simulink model "Proposed DTC"  (R2022a)
settings: Solver=ode1  StartTime=0.0  StopTime=Inf  FixedStep=Ts  RelTol=1e-3  EnableMultiTasking=on
PostLoadFcn:
  | , if any(exist('dsrtsu_mdlpostloadfcn', 'file') ~= 0), dsrtsu_mdlpostloadfcn('Execute', bdroot); end,
InitFcn:
  | , if any(exist('rtifpga_mdlclblib', 'file') ~= 0), rtifpga_mdlclblib('Init', bdroot); end,
undefined symbols (not defined in the file): P, Ts
libraries: rtilib1104 x15, rtitasklib x1
(part 2 of 2)

== matlab function Proposed DTC/Controller/MATLAB Function2 ==
  data: del_psi input; V output; del_T input; n input; psi_s1 input; is_1 input; psi_s_ref input; T_ref input; Vdc input; Ts input; w input; Dfinal output
function [V,Dfinal] = fcn(del_psi,del_T,n,psi_s1,is_1,psi_s_ref,T_ref,Vdc,Ts,w)
Dfinal=1;
T_max=1; T_min=-1;
psi_max=0.01; psi_min=-0.01;
Ls=0.022;
psi_r=0.5;
V=1;
V1=2/5*Vdc*(1.6180+1j*0);
V2=2/5*Vdc*(1.3090+1j*0.9511);
V3=2/5*Vdc*(0.5+1j*1.5390);
V4=2/5*Vdc*(-0.5+1j*1.5390);
V5=2/5*Vdc*(-1.3090+1j*0.9511);
V6=2/5*Vdc*(-1.6180+1j*0);
V7=2/5*Vdc*(-1.3090-1j*0.9511);
V8=2/5*Vdc*(-0.5-1j*1.5390);
V9=2/5*Vdc*(0.5-1j*1.5390);
V10=2/5*Vdc*(1.3090-1j*0.9511);
V11=2/5*Vdc*(1+1j*0);
V12=2/5*Vdc*(0.8090+1j*0.5878);
V13=2/5*Vdc*(0.3090+1j*0.9511);
V14=2/5*Vdc*(-0.3090+1j*0.9511);
V15=2/5*Vdc*(-0.8090+1j*0.5878);
V16=2/5*Vdc*(-1+1j*0);
V17=2/5*Vdc*(-0.8090-1j*0.5878);
V18=2/5*Vdc*(-0.3090-1j*0.9511);
V19=2/5*Vdc*(0.3090-1j*0.9511);
V20=2/5*Vdc*(0.8090-1j*0.5878);
V21=2/5*Vdc*(0.6180+1j*0);
V22=2/5*Vdc*(0.5+1j*0.3633);
V23=2/5*Vdc*(0.1910+1j*0.5878);
V24=2/5*Vdc*(-0.1910+1j*0.5878);
V25=2/5*Vdc*(-0.5+1j*0.3633);
V26=2/5*Vdc*(-0.6180+1j*0);
V27=2/5*Vdc*(-0.5-1j*0.3633);
V28=2/5*Vdc*(-0.1910-1j*0.5878);
V29=2/5*Vdc*(0.1910-1j*0.5878);
V30=2/5*Vdc*(0.5-1j*0.3633);
V31=0;
v=[V1 V2 V3 V4 V5 V6 V7 V8 V9 V10 V11 V12 V13 V14 V15 V16 V17 V18 V19 V20 V21 V22 V23 V24 V25 V26 V27 V28 V29 V30 V31];
% states=[1 1 0 0 1;
%         1 1 0 0 0;
%         1 1 1 0 0;
%         0 1 1 0 0;
%         0 1 1 1 0;
%         0 0 1 1 0;
%         0 0 1 1 1;
%         0 0 0 1 1;
%         1 0 0 1 1;
%         1 0 0 0 1;
%         1 0 0 0 0;
%         1 1 1 0 1;
%         0 1 0 0 0;
%         1 1 1 1 0;
%         0 0 1 0 0;
%         0 1 1 1 1;
%         0 0 0 1 0;
%         1 0 1 1 1;
%         0 0 0 0 1;
%         1 1 0 1 1;
%         0 1 0 0 1;
%         1 1 0 1 0;
%         1 0 1 0 0;
%         0 1 1 0 1;
%         0 1 0 1 0;
%         1 0 1 1 0;
%         0 0 1 0 1;
%         0 1 0 1 1;
%         1 0 0 1 0;
%         1 0 1 0 1;
%         0 0 0 0 0];
VT=0;Vpsi=0;
kk=0;
persistent dec k D_psi D_T x y 
if isempty(dec), dec = 0; end
if isempty(k), k = 0; end
if isempty(D_psi), D_psi = 0; end
if isempty(D_T), D_T = 0; end
if isempty(x), x = 31; end
if isempty(y), y = 31; end

if del_T>T_max
    del_T=1;
elseif del_T<T_min
    del_T=-1;
else
    del_T=0;
end
if del_psi>psi_max
    del_psi=1;
elseif del_psi<psi_min
    del_psi=-1;
else
    del_psi=0;
end
%     D=1;
if abs(w)>157.07
    D=abs(w)/314;
else
    D=0.5;
end
% High speed of operation
if((abs(w)>=0&&abs(w)<=314))
if dec==0
    if del_T==1
        if n==1 || n==2
            VT=v(4);x=4;
        elseif n==3 || n==4
            VT=v(5);x=5;
        elseif n==5 || n==6
            VT=v(6);x=6;
        elseif n==7 || n==8
            VT=v(7);x=7;
        elseif n==9 || n==10
            VT=v(8);x=8;
        elseif n==11 || n==12
            VT=v(9);x=9;
        elseif n==13 || n==14
            VT=v(10);x=10;
        elseif n==15 || n==16
            VT=v(1);x=1;
        elseif n==17 || n==18
            VT=v(2);x=2;
        elseif n==19 || n==20
            VT=v(3);x=3;
        end
    elseif del_T==-1
        if n==1 || n==2
            VT=v(9);x=9;
        elseif n==3 || n==4
            VT=v(10);x=10;
        elseif n==5 || n==6
            VT=v(1);x=1;
        elseif n==7 || n==8
            VT=v(2);x=2;
        elseif n==9 || n==10
            VT=v(3);x=3;
        elseif n==11 || n==12
            VT=v(4);x=4;
        elseif n==13 || n==14
            VT=v(5);x=5;
        elseif n==15 || n==16
            VT=v(6);x=6;
        elseif n==17 || n==18
            VT=v(7);x=7;
        elseif n==19 || n==20
            VT=v(8);x=8;
        end
    end
    if del_psi==1
        if n==2 || n==3
            Vpsi=v(2);y=2;
            VT=v(4);x=4;
            if del_T==-1
                VT=v(10);x=10;
            end
        elseif n==4 || n==5
            Vpsi=v(3);y=3;
            VT=v(5);x=5;
            if del_T==-1
                VT=v(1);x=1;
            end
        elseif n==6 || n==7
            Vpsi=v(4);y=4;
            VT=v(6);x=6;
            if del_T==-1
                VT=v(2);x=2;
            end
        elseif n==8 || n==9
            Vpsi=v(5);y=5;
            VT=v(7);x=7;
            if del_T==-1
                VT=v(3);x=3;
            end
        elseif n==10 || n==11
            Vpsi=v(6);y=6;
            VT=v(8);x=8;
            if del_T==-1
                VT=v(4);x=4;
            end
        elseif n==12 || n==13
            Vpsi=v(7);y=7;
            VT=v(9);x=9;
            if del_T==-1
                VT=v(5);x=5;
            end
        elseif n==14 || n==15
            Vpsi=v(8);y=8;
            VT=v(10);x=10;
            if del_T==-1
                VT=v(6);x=6;
            end
        elseif n==16 || n==17
            Vpsi=v(9);y=9;
            VT=v(1);x=1;
            if del_T==-1
                VT=v(7);x=7;
            end
        elseif n==18 || n==19
            Vpsi=v(10);y=10;
            VT=v(2);x=2;
            if del_T==-1
                VT=v(8);x=8;
            end
        elseif n==20 || n==1
            Vpsi=v(1);y=1;
            VT=v(3);x=3;
            if del_T==-1
                VT=v(9);x=9;
            end
        end
    elseif del_psi==-1
        if n==2 || n==3
            Vpsi=v(7);y=7;
            VT=v(5);x=5;
            if del_T==-1
                VT=v(9);x=9;
            end
        elseif n==4 || n==5
            Vpsi=v(8);y=8;
            VT=v(6);x=6;
            if del_T==-1
                VT=v(10);x=10;
            end
        elseif n==6 || n==7
            Vpsi=v(9);y=9;
            VT=v(7);x=7;
            if del_T==-1
                VT=v(1);x=1;
            end
        elseif n==8 || n==9
            Vpsi=v(10);y=10;
            VT=v(8);x=8;
            if del_T==-1
                VT=v(2);x=2;
            end
        elseif n==10 || n==11
            Vpsi=v(1);y=1;
            VT=v(9);x=9;
            if del_T==-1
                VT=v(3);x=3;
            end
        elseif n==12 || n==13
            Vpsi=v(2);y=2;
            VT=v(10);x=10;
            if del_T==-1
                VT=v(4);x=4;
            end
        elseif n==14 || n==15
            Vpsi=v(3);y=3;
            VT=v(1);x=1;
            if del_T==-1
                VT=v(5);x=5;
            end
         elseif n==16 || n==17
            Vpsi=v(4);y=4;
            VT=v(2);x=2;
            if del_T==-1
                VT=v(6);x=6;
            end
         elseif n==18 || n==19
            Vpsi=v(5);y=5;
            VT=v(3);x=3;
            if del_T==-1
                VT=v(7);x=7;
            end
         elseif n==20 || n==1
            Vpsi=v(6);y=6;
            VT=v(4);x=4;
            if del_T==-1
                VT=v(8);x=8;
            end
        end
    elseif del_psi==0
        y=x;
    end
    if del_T==0
        VT=0;Vpsi=0;x=31;y=31;
    end    
    M=abs(VT)*Ts*sin(angle(VT)-angle(psi_s1));    
    Q=Ls*(T_ref/(5*psi_r)-abs(is_1)*sin(angle(is_1)-angle(psi_s1)));    
    if del_T==0
        D_psi=0;
        D_T=0;
    end
    dec=1;
    if del_psi==0
        D_T=0.5*Q/M;        
        D_psi=D_T;
    else
        D_T=D;
        kk=1;
        k=1;
    end
    V=x;
    Dfinal=D_T;
end
k=k+1;
if k==2
    k=0;
    dec=0;
end
if dec==0 && kk==0
    if del_T==1
        if n==1 || n==2
            VT=v(4);x=4;
        elseif n==3 || n==4
            VT=v(5);x=5;
        elseif n==5 || n==6
            VT=v(6);x=6;
        elseif n==7 || n==8
            VT=v(7);x=7;
        elseif n==9 || n==10
            VT=v(8);x=8;
        elseif n==11 || n==12
            VT=v(9);x=9;
        elseif n==13 || n==14
            VT=v(10);x=10;
        elseif n==15 || n==16
            VT=v(1);x=1;
        elseif n==17 || n==18
            VT=v(2);x=2;
        elseif n==19 || n==20
            VT=v(3);x=3;
        end
    elseif del_T==-1
        if n==1 || n==2
            VT=v(9);x=9;
        elseif n==3 || n==4
            VT=v(10);x=10;
        elseif n==5 || n==6
            VT=v(1);x=1;
        elseif n==7 || n==8
            VT=v(2);x=2;
        elseif n==9 || n==10
            VT=v(3);x=3;
        elseif n==11 || n==12
            VT=v(4);x=4;
        elseif n==13 || n==14
            VT=v(5);x=5;
        elseif n==15 || n==16
            VT=v(6);x=6;
        elseif n==17 || n==18
            VT=v(7);x=7;
        elseif n==19 || n==20
            VT=v(8);x=8;
        end
    end

    if del_psi==1
        if n==2 || n==3
            Vpsi=v(2);k=0;
        elseif n==4 || n==5
            Vpsi=v(3);k=0;
        elseif n==6 || n==7
            Vpsi=v(4);k=0;
        elseif n==8 || n==9
            Vpsi=v(5);k=0;
        elseif n==10 || n==11
            Vpsi=v(6);k=0;
        elseif n==12 || n==13
            Vpsi=v(7);k=0;
        elseif n==14 || n==15
            Vpsi=v(8);k=0;
        elseif n==16 || n==17
            Vpsi=v(9);k=0;
        elseif n==18 || n==19
            Vpsi=v(10);k=0;
        elseif n==20 || n==1
            Vpsi=v(1);k=0;    
        end
    elseif del_psi==0
        if n==2 || n==3
            Vpsi=v(7);k=0;
        elseif n==4 || n==5
            Vpsi=v(8);k=0;
        elseif n==6 || n==7
            Vpsi=v(9);k=0;
        elseif n==8 || n==9
            Vpsi=v(10);k=0;
        elseif n==10 || n==11
            Vpsi=v(1);k=0;
        elseif n==12 || n==13
            Vpsi=v(2);k=0;
        elseif n==14 || n==15
            Vpsi=v(3);k=0;
        elseif n==16 || n==17
            Vpsi=v(4);k=0;
        elseif n==18 || n==19
            Vpsi=v(5);k=0;
        elseif n==20 || n==1
            Vpsi=v(6);k=0;
        end
    end
    if del_T==0
        VT=0;Vpsi=0;x=31;
    end
    A=abs(VT)*Ts*cos(angle(VT)-angle(psi_s1));
    B=abs(Vpsi)*Ts*cos(angle(Vpsi)-angle(psi_s1));
    M=abs(VT)*Ts*sin(angle(VT)-angle(psi_s1));
    N=abs(Vpsi)*Ts*sin(angle(Vpsi)-angle(psi_s1));
    K=psi_s_ref-abs(psi_s1);
    Q=Ls*(T_ref/(5*psi_r)-abs(is_1)*sin(angle(is_1)-angle(psi_s1)));
    V=y;
    Dfinal=D_psi;
end
% Medium speed of operation
% elseif(abs(w)>100 && abs(w)<=200)
% if dec==0
%     if del_T==1
%         if n==1 || n==2
%             VT=v(14);x=14;
%         elseif n==3 || n==4
%             VT=v(15);x=15;
%         elseif n==5 || n==6
%             VT=v(16);x=16;
%         elseif n==7 || n==8
%             VT=v(17);x=17;
%         elseif n==9 || n==10
%             VT=v(18);x=18;
%         elseif n==11 || n==12
%             VT=v(19);x=19;
%         elseif n==13 || n==14
%             VT=v(20);x=20;
%         elseif n==15 || n==16
%             VT=v(11);x=11;
%         elseif n==17 || n==18
%             VT=v(12);x=12;
%         elseif n==19 || n==20
%             VT=v(13);x=13;
%         end
%     elseif del_T==-1
%         if n==1 || n==2
%             VT=v(19);x=19;
%         elseif n==3 || n==4
%             VT=v(20);x=20;
%         elseif n==5 || n==6
%             VT=v(11);x=11;
%         elseif n==7 || n==8
%             VT=v(12);x=12;
%         elseif n==9 || n==10
%             VT=v(13);x=13;
%         elseif n==11 || n==12
%             VT=v(14);x=14;
%         elseif n==13 || n==14
%             VT=v(15);x=15;
%         elseif n==15 || n==16
%             VT=v(16);x=16;
%         elseif n==17 || n==18
%             VT=v(17);x=17;
%         elseif n==19 || n==20
%             VT=v(18);x=18;
%         end
%     end
%     if del_psi==1
%         if n==2 || n==3
%             Vpsi=v(12);y=12;
%             VT=v(14);x=14;
%             if del_T==-1
%                 VT=v(20);x=20;
%             end
%         elseif n==4 || n==5
%             Vpsi=v(13);y=13;
%             VT=v(15);x=15;
%             if del_T==-1
%                 VT=v(11);x=11;
%             end
%         elseif n==6 || n==7
%             Vpsi=v(14);y=14;
%             VT=v(16);x=16;
%             if del_T==-1
%                 VT=v(12);x=12;
%             end
%         elseif n==8 || n==9
%             Vpsi=v(15);y=15;
%             VT=v(17);x=17;
%             if del_T==-1
%                 VT=v(13);x=13;
%             end
%         elseif n==10 || n==11
%             Vpsi=v(16);y=16;
%             VT=v(18);x=18;
%             if del_T==-1
%                 VT=v(14);x=14;
%             end
%         elseif n==12 || n==13
%             Vpsi=v(17);y=17;
%             VT=v(19);x=19;
%             if del_T==-1
%                 VT=v(15);x=15;
%             end
%         elseif n==14 || n==15
%             Vpsi=v(18);y=18;
%             VT=v(20);x=20;
%             if del_T==-1
%                 VT=v(16);x=16;
%             end
%         elseif n==16 || n==17
%             Vpsi=v(19);y=19;
%             VT=v(11);x=11;
%             if del_T==-1
%                 VT=v(17);x=17;
%             end
%         elseif n==18 || n==19
%             Vpsi=v(20);y=20;
%             VT=v(12);x=12;
%             if del_T==-1
%                 VT=v(18);x=18;
%             end
%         elseif n==20 || n==1
%             Vpsi=v(11);y=11;
%             VT=v(13);x=13;
%             if del_T==-1
%                 VT=v(19);x=19;
%             end
%         end
%     elseif del_psi==-1
%         if n==2 || n==3
%             Vpsi=v(17);y=17;
%             VT=v(15);x=15;
%             if del_T==-1
%                 VT=v(19);x=19;
%             end
%         elseif n==4 || n==5
%             Vpsi=v(18);y=18;
%             VT=v(16);x=16;
%             if del_T==-1
%                 VT=v(20);x=20;
%             end
%         elseif n==6 || n==7
%             Vpsi=v(19);y=19;
%             VT=v(17);x=17;
%             if del_T==-1
%                 VT=v(11);x=11;
%             end
%         elseif n==8 || n==9
%             Vpsi=v(20);y=20;
%             VT=v(18);x=18;
%             if del_T==-1
%                 VT=v(12);x=12;
%             end
%         elseif n==10 || n==11
%             Vpsi=v(11);y=11;
%             VT=v(19);x=19;
%             if del_T==-1
%                 VT=v(13);x=13;
%             end
%         elseif n==12 || n==13
%             Vpsi=v(12);y=12;
%             VT=v(20);x=20;
%             if del_T==-1
%                 VT=v(14);x=14;
%             end
%         elseif n==14 || n==15
%             Vpsi=v(13);y=13;
%             VT=v(11);x=11;
%             if del_T==-1
%                 VT=v(15);x=15;
%             end
%          elseif n==16 || n==17
%             Vpsi=v(14);y=14;
%             VT=v(12);x=12;
%             if del_T==-1
%                 VT=v(16);x=16;
%             end
%          elseif n==18 || n==19
%             Vpsi=v(15);y=15;
%             VT=v(13);x=13;
%             if del_T==-1
%                 VT=v(17);x=17;
%             end
%          elseif n==20 || n==1
%             Vpsi=v(16);y=16;
%             VT=v(14);x=14;
%             if del_T==-1
%                 VT=v(18);x=18;
%             end
%         end
%     elseif del_psi==0
%         y=x;
%     end
%     if del_T==0
%         VT=0;Vpsi=0;x=31;y=31;
%     end    
%     M=abs(VT)*Ts*sin(angle(VT)-angle(psi_s1));    
%      Q=Ls*(T_ref/(5*psi_r)-abs(is_1)*sin(angle(is_1)-angle(psi_s1)));   
%     if del_T==0
%         D_psi=0;
%         D_T=0;
%     end
%     dec=1;
%     if del_psi==0
%         D_T=0.5*Q/M;        
%         D_psi=D_T;
%     else
%         D_T=D;
%         kk=1;
%         k=1;
%     end
%     V=x;
%     Dfinal=D_T;
% end
% k=k+1;
% if k==2
%     k=0;
%     dec=0;
% end
% if dec==0 && kk==0
%     if del_T==1
%         if n==1 || n==2
%             VT=v(14);x=14;
%         elseif n==3 || n==4
%             VT=v(15);x=15;
%         elseif n==5 || n==6
%             VT=v(16);x=16;
%         elseif n==7 || n==8
%             VT=v(17);x=17;
%         elseif n==9 || n==10
%             VT=v(18);x=18;
%         elseif n==11 || n==12
%             VT=v(19);x=19;
%         elseif n==13 || n==14
%             VT=v(20);x=20;
%         elseif n==15 || n==16
%             VT=v(11);x=11;
%         elseif n==17 || n==18
%             VT=v(12);x=12;
%         elseif n==19 || n==20
%             VT=v(13);x=13;
%         end
%     elseif del_T==-1
%         if n==1 || n==2
%             VT=v(19);x=19;
%         elseif n==3 || n==4
%             VT=v(20);x=20;
%         elseif n==5 || n==6
%             VT=v(11);x=11;
%         elseif n==7 || n==8
%             VT=v(12);x=12;
%         elseif n==9 || n==10
%             VT=v(13);x=13;
%         elseif n==11 || n==12
%             VT=v(14);x=14;
%         elseif n==13 || n==14
%             VT=v(15);x=15;
%         elseif n==15 || n==16
%             VT=v(16);x=16;
%         elseif n==17 || n==18
%             VT=v(17);x=17;
%         elseif n==19 || n==20
%             VT=v(18);x=18;
%         end
%     end
% 
%     if del_psi==1
%         if n==2 || n==3
%             Vpsi=v(12);k=0;
%         elseif n==4 || n==5
%             Vpsi=v(13);k=0;
%         elseif n==6 || n==7
%             Vpsi=v(14);k=0;
%         elseif n==8 || n==9
%             Vpsi=v(15);k=0;
%         elseif n==10 || n==11
%             Vpsi=v(16);k=0;
%         elseif n==12 || n==13
%             Vpsi=v(17);k=0;
%         elseif n==14 || n==15
%             Vpsi=v(18);k=0;
%         elseif n==16 || n==17
%             Vpsi=v(19);k=0;
%         elseif n==18 || n==19
%             Vpsi=v(20);k=0;
%         elseif n==20 || n==1
%             Vpsi=v(11);k=0;    
%         end
%     elseif del_psi==0
%         if n==2 || n==3
%             Vpsi=v(17);k=0;
%         elseif n==4 || n==5
%             Vpsi=v(18);k=0;
%         elseif n==6 || n==7
%             Vpsi=v(19);k=0;
%         elseif n==8 || n==9
%             Vpsi=v(20);k=0;
%         elseif n==10 || n==11
%             Vpsi=v(11);k=0;
%         elseif n==12 || n==13
%             Vpsi=v(12);k=0;
%         elseif n==14 || n==15
%             Vpsi=v(13);k=0;
%         elseif n==16 || n==17
%             Vpsi=v(14);k=0;
%         elseif n==18 || n==19
%             Vpsi=v(15);k=0;
%         elseif n==20 || n==1
%             Vpsi=v(16);k=0;
%         end
%     end
%     if del_T==0
%         VT=0;Vpsi=0;x=31;
%     end
%     A=abs(VT)*Ts*cos(angle(VT)-angle(psi_s1));
%     B=abs(Vpsi)*Ts*cos(angle(Vpsi)-angle(psi_s1));
%     M=abs(VT)*Ts*sin(angle(VT)-angle(psi_s1));
%     N=abs(Vpsi)*Ts*sin(angle(Vpsi)-angle(psi_s1));
%     K=psi_s_ref-abs(psi_s1);
%     Q=Ls*(T_ref/(5*psi_r)-abs(is_1)*sin(angle(is_1)-angle(psi_s1)));
%     V=y;
%     Dfinal=D_psi;
% end    
% % Low speed of operation
% elseif(abs(w)>=0 && abs(w)<=100)
% if dec==0
%     if del_T==1
%         if n==1 || n==2
%             VT=v(24);x=24;
%         elseif n==3 || n==4
%             VT=v(25);x=25;
%         elseif n==5 || n==6
%             VT=v(26);x=26;
%         elseif n==7 || n==8
%             VT=v(27);x=27;
%         elseif n==9 || n==10
%             VT=v(28);x=28;
%         elseif n==11 || n==12
%             VT=v(29);x=29;
%         elseif n==13 || n==14
%             VT=v(30);x=30;
%         elseif n==15 || n==16
%             VT=v(21);x=21;
%         elseif n==17 || n==18
%             VT=v(22);x=22;
%         elseif n==19 || n==20
%             VT=v(23);x=23;
%         end
%     elseif del_T==-1
%         if n==1 || n==2
%             VT=v(29);x=29;
%         elseif n==3 || n==4
%             VT=v(30);x=30;
%         elseif n==5 || n==6
%             VT=v(21);x=21;
%         elseif n==7 || n==8
%             VT=v(22);x=22;
%         elseif n==9 || n==10
%             VT=v(23);x=23;
%         elseif n==11 || n==12
%             VT=v(24);x=24;
%         elseif n==13 || n==14
%             VT=v(25);x=25;
%         elseif n==15 || n==16
%             VT=v(26);x=26;
%         elseif n==17 || n==18
%             VT=v(27);x=27;
%         elseif n==19 || n==20
%             VT=v(28);x=28;
%         end
%     end
%     if del_psi==1
%         if n==2 || n==3
%             Vpsi=v(22);y=22;
%             VT=v(24);x=24;
%             if del_T==-1
%                 VT=v(30);x=30;
%             end
%         elseif n==4 || n==5
%             Vpsi=v(23);y=23;
%             VT=v(25);x=25;
%             if del_T==-1
%                 VT=v(21);x=21;
%             end
%         elseif n==6 || n==7
%             Vpsi=v(24);y=24;
%             VT=v(26);x=26;
%             if del_T==-1
%                 VT=v(22);x=22;
%             end
%         elseif n==8 || n==9
%             Vpsi=v(25);y=25;
%             VT=v(27);x=27;
%             if del_T==-1
%                 VT=v(23);x=23;
%             end
%         elseif n==10 || n==11
%             Vpsi=v(26);y=26;
%             VT=v(28);x=28;
%             if del_T==-1
%                 VT=v(24);x=24;
%             end
%         elseif n==12 || n==13
%             Vpsi=v(27);y=27;
%             VT=v(29);x=29;
%             if del_T==-1
%                 VT=v(25);x=25;
%             end
%         elseif n==14 || n==15
%             Vpsi=v(28);y=28;
%             VT=v(30);x=30;
%             if del_T==-1
%                 VT=v(26);x=26;
%             end
%         elseif n==16 || n==17
%             Vpsi=v(29);y=29;
%             VT=v(21);x=21;
%             if del_T==-1
%                 VT=v(27);x=27;
%             end
%         elseif n==18 || n==19
%             Vpsi=v(30);y=30;
%             VT=v(22);x=22;
%             if del_T==-1
%                 VT=v(28);x=28;
%             end
%         elseif n==20 || n==1
%             Vpsi=v(21);y=21;
%             VT=v(23);x=23;
%             if del_T==-1
%                 VT=v(29);x=29;
%             end
%         end
%     elseif del_psi==-1
%         if n==2 || n==3
%             Vpsi=v(27);y=27;
%             VT=v(25);x=25;
%             if del_T==-1
%                 VT=v(29);x=29;
%             end
%         elseif n==4 || n==5
%             Vpsi=v(28);y=28;
%             VT=v(26);x=26;
%             if del_T==-1
%                 VT=v(30);x=30;
%             end
%         elseif n==6 || n==7
%             Vpsi=v(29);y=29;
%             VT=v(27);x=27;
%             if del_T==-1
%                 VT=v(21);x=21;
%             end
%         elseif n==8 || n==9
%             Vpsi=v(30);y=30;
%             VT=v(28);x=28;
%             if del_T==-1
%                 VT=v(22);x=22;
%             end
%         elseif n==10 || n==11
%             Vpsi=v(21);y=21;
%             VT=v(29);x=29;
%             if del_T==-1
%                 VT=v(23);x=23;
%             end
%         elseif n==12 || n==13
%             Vpsi=v(22);y=22;
%             VT=v(30);x=30;
%             if del_T==-1
%                 VT=v(24);x=24;
%             end
%         elseif n==14 || n==15
%             Vpsi=v(23);y=23;
%             VT=v(21);x=21;
%             if del_T==-1
%                 VT=v(25);x=25;
%             end
%          elseif n==16 || n==17
%             Vpsi=v(24);y=24;
%             VT=v(22);x=22;
%             if del_T==-1
%                 VT=v(26);x=26;
%             end
%          elseif n==18 || n==19
%             Vpsi=v(25);y=25;
%             VT=v(23);x=23;
%             if del_T==-1
%                 VT=v(27);x=27;
%             end
%          elseif n==20 || n==1
%             Vpsi=v(26);y=26;
%             VT=v(24);x=24;
%             if del_T==-1
%                 VT=v(28);x=28;
%             end
%         end
%     elseif del_psi==0
%         y=x;
%     end
%     if del_T==0
%         VT=0;Vpsi=0;x=31;y=31;
%     end    
%     M=abs(VT)*Ts*sin(angle(VT)-angle(psi_s1));    
%      Q=Ls*(T_ref/(5*psi_r)-abs(is_1)*sin(angle(is_1)-angle(psi_s1)));   
%     if del_T==0
%         D_psi=0;
%         D_T=0;
%     end
%     dec=1;
%     if del_psi==0
%         D_T=0.5*Q/M;        
%         D_psi=D_T;
%     else
%         D_T=D;
%         kk=1;
%         k=1;
%     end
%      V=x;
%     Dfinal=D_T;
% end
% k=k+1;
% if k==2
%     k=0;
%     dec=0;
% end
% if dec==0 && kk==0
%     if del_T==1
%         if n==1 || n==2
%             VT=v(24);x=24;
%         elseif n==3 || n==4
%             VT=v(25);x=25;
%         elseif n==5 || n==6
%             VT=v(26);x=26;
%         elseif n==7 || n==8
%             VT=v(27);x=27;
%         elseif n==9 || n==10
%             VT=v(28);x=28;
%         elseif n==11 || n==12
%             VT=v(29);x=29;
%         elseif n==13 || n==14
%             VT=v(30);x=30;
%         elseif n==15 || n==16
%             VT=v(21);x=21;
%         elseif n==17 || n==18
%             VT=v(22);x=22;
%         elseif n==19 || n==20
%             VT=v(23);x=23;
%         end
%     elseif del_T==-1
%         if n==1 || n==2
%             VT=v(29);x=29;
%         elseif n==3 || n==4
%             VT=v(30);x=30;
%         elseif n==5 || n==6
%             VT=v(21);x=21;
%         elseif n==7 || n==8
%             VT=v(22);x=22;
%         elseif n==9 || n==10
%             VT=v(23);x=23;
%         elseif n==11 || n==12
%             VT=v(24);x=24;
%         elseif n==13 || n==14
%             VT=v(25);x=25;
%         elseif n==15 || n==16
%             VT=v(26);x=26;
%         elseif n==17 || n==18
%             VT=v(27);x=27;
%         elseif n==19 || n==20
%             VT=v(28);x=28;
%         end
%     end
% 
%     if del_psi==1
%         if n==2 || n==3
%             Vpsi=v(22);k=0;
%         elseif n==4 || n==5
%             Vpsi=v(23);k=0;
%         elseif n==6 || n==7
%             Vpsi=v(24);k=0;
%         elseif n==8 || n==9
%             Vpsi=v(25);k=0;
%         elseif n==10 || n==11
%             Vpsi=v(26);k=0;
%         elseif n==12 || n==13
%             Vpsi=v(27);k=0;
%         elseif n==14 || n==15
%             Vpsi=v(28);k=0;
%         elseif n==16 || n==17
%             Vpsi=v(29);k=0;
%         elseif n==18 || n==19
%             Vpsi=v(30);k=0;
%         elseif n==20 || n==1
%             Vpsi=v(21);k=0;    
%         end
%     elseif del_psi==0
%         if n==2 || n==3
%             Vpsi=v(27);k=0;
%         elseif n==4 || n==5
%             Vpsi=v(28);k=0;
%         elseif n==6 || n==7
%             Vpsi=v(29);k=0;
%         elseif n==8 || n==9
%             Vpsi=v(30);k=0;
%         elseif n==10 || n==11
%             Vpsi=v(21);k=0;
%         elseif n==12 || n==13
%             Vpsi=v(22);k=0;
%         elseif n==14 || n==15
%             Vpsi=v(23);k=0;
%         elseif n==16 || n==17
%             Vpsi=v(24);k=0;
%         elseif n==18 || n==19
%             Vpsi=v(25);k=0;
%         elseif n==20 || n==1
%             Vpsi=v(26);k=0;
%         end
%     end
%     if del_T==0
%         VT=0;Vpsi=0;x=31;
%     end
%     A=abs(VT)*Ts*cos(angle(VT)-angle(psi_s1));
%     B=abs(Vpsi)*Ts*cos(angle(Vpsi)-angle(psi_s1));
%     M=abs(VT)*Ts*sin(angle(VT)-angle(psi_s1));
%     N=abs(Vpsi)*Ts*sin(angle(Vpsi)-angle(psi_s1));
%     K=psi_s_ref-abs(psi_s1);
%     Q=Ls*(T_ref/(5*psi_r)-abs(is_1)*sin(angle(is_1)-angle(psi_s1)));
%       V=y;
%     Dfinal=D_psi;
% end    
end 
if(Dfinal>1)
    Dfinal=1;
end
%dec1=dec;
end

== matlab function Proposed DTC/MATLAB Function1 ==
  data: ia input; id1 output; ib input; ic input; id input; ie input; th input; iq1 output; id3 output; iq3 output
function [id1,iq1,id3,iq3]= fcn(ia,ib,ic,id,ie,th)
id1=(2/5)*(ia+(ib*cos(th))+(ic*cos(2*th))+(id*cos(3*th))+(ie*cos(4*th)));
iq1=(2/5)*(((ib*sin(th))+(ic*sin(2*th))+(id*sin(3*th))+(ie*sin(4*th))));
id3=(2/5)*(ia+(ib*cos(3*th))+(ic*cos(6*th))+(id*cos(9*th))+(ie*cos(12*th)));
iq3=(2/5)*(((ib*sin(3*th))+(ic*sin(6*th))+(id*sin(9*th))+(ie*sin(12*th))));
end

== matlab function Proposed DTC/Controller/Subsystem1/States ==
  data: vv input; Sa output; Sb output; Sc output; Sd output; Se output

function [Sa,Sb,Sc,Sd,Se] = fcn(vv)
    if(vv==0)
    Sa=0;
    Sb=0;
    Sc=0; 
    Sd=0;
    Se=0;
    elseif(vv==1)
    Sa=1;
    Sb=1;
    Sc=0; 
    Sd=0;
    Se=1;
    elseif(vv==2)
    Sa=1;
    Sb=1;
    Sc=0;
    Sd=0;
    Se=0;
    elseif(vv==3)
    Sa=1;
    Sb=1;
    Sc=1;
    Sd=0;
    Se=0;
    elseif(vv==4)
    Sa=0;
    Sb=1;
    Sc=1;
    Sd=0;
    Se=0;
    elseif(vv==5)
    Sa=0;
    Sb=1;
    Sc=1;
    Sd=1;
    Se=0;
    elseif(vv==6)
    Sa=0;
    Sb=0;
    Sc=1;
    Sd=1;
    Se=0;
    elseif(vv==7)
    Sa=0;
    Sb=0;
    Sc=1;
    Sd=1;
    Se=1;
    elseif(vv==8)
    Sa=0;
    Sb=0;
    Sc=0;
    Sd=1;
    Se=1;
    elseif(vv==9)
    Sa=1;
    Sb=0;
    Sc=0;
    Sd=1;
    Se=1;
    elseif(vv==10)
    Sa=1;
    Sb=0;
    Sc=0;
    Sd=0;
    Se=1;
    elseif(vv==11)
    Sa=1;
    Sb=0;
    Sc=0;
    Sd=0;
    Se=0;
    elseif(vv==12)
    Sa=1;
    Sb=1;
    Sc=1;
    Sd=0;
    Se=1;
    elseif(vv==13)
    Sa=0;
    Sb=1;
    Sc=0;
    Sd=0;
    Se=0;
    elseif(vv==14)
    Sa=1;
    Sb=1;
    Sc=1;
    Sd=1;
    Se=0;
    elseif(vv==15)
    Sa=0;
    Sb=0;
    Sc=1;
    Sd=0;
    Se=0;
    elseif(vv==16)
    Sa=0;
    Sb=1;
    Sc=1;
    Sd=1;
    Se=1;
    elseif(vv==17)
    Sa=0;
    Sb=0;
    Sc=0;
    Sd=1;
    Se=0;
    elseif(vv==18)
    Sa=1;
    Sb=0;
    Sc=1;
    Sd=1;
    Se=1;
    elseif(vv==19)
    Sa=0;
    Sb=0;
    Sc=0;
    Sd=0;
    Se=1;
    elseif(vv==20)
    Sa=1;
    Sb=1;
    Sc=0;
    Sd=1;
    Se=1;
    elseif(vv==21)
    Sa=0;
    Sb=1;
    Sc=0;
    Sd=0;
    Se=1;
    elseif(vv==22)
    Sa=1;
    Sb=1;
    Sc=0;
    Sd=1;
    Se=0;
    elseif(vv==23)
    Sa=1;
    Sb=0;
    Sc=1;
    Sd=0;
    Se=0;
    elseif(vv==24)
    Sa=0;
    Sb=1;
    Sc=1;
    Sd=0;
    Se=1;
    elseif(vv==25)
    Sa=0;
    Sb=1;
    Sc=0;
    Sd=1;
    Se=0;
    elseif(vv==26)
    Sa=1;
    Sb=0;
    Sc=1;
    Sd=1;
    Se=0;
    elseif(vv==27)
    Sa=0;
    Sb=0;
    Sc=1;
    Sd=0;
    Se=1;
    elseif(vv==28)
    Sa=0;
    Sb=1;
    Sc=0;
    Sd=1;
    Se=1;
    elseif(vv==29)
    Sa=1;
    Sb=0;
    Sc=0;
    Sd=1;
    Se=0;
    else
    Sa=1;
    Sb=0;
    Sc=1;
    Sd=0;
    Se=1;
    end

== matlab function Proposed DTC/Controller/5Phase SECTOR SELECTION radians2 ==
  data: Sa input; DSa output; Sb input; Sc input; Sd input; Se input; D input; DSb output; DSc output; DSd output; DSe output
function [DSa,DSb,DSc,DSd,DSe] = fcn(Sa,Sb,Sc,Sd,Se,D)
DSa=D*Sa;
DSb=D*Sb;
DSc=D*Sc;
DSd=D*Sd;
DSe=D*Se;
end

== matlab function Proposed DTC/Controller/5Phase SECTOR SELECTION radians1 ==
  data: theta input; sector output
function sector = fcn(theta)
if(theta>-pi/10 && theta<=pi/10)
    sector=1;
elseif(theta>pi/10 && theta<=3*pi/10)
    sector=2;
elseif(theta>3*pi/10 && theta<=pi/2)
    sector=3;
elseif(theta>pi/2 && theta<=7*pi/10)
    sector=4;
elseif(theta>7*pi/10 && theta<=9*pi/10)
    sector=5;
elseif(theta>-9*pi/10 && theta<=-7*pi/10)
    sector=7;
elseif(theta>-7*pi/10 && theta<=-pi/2)
    sector=8;
elseif(theta>-pi/2 && theta<=-3*pi/10)
    sector=9;
elseif(theta>-3*pi/10 && theta<=-pi/10)
    sector=10;        
else
    sector=6;
end

== matlab function Proposed DTC/Controller/Torque & flux estimator ==
  data: psi_s_mag output; alfa output; Te output; i_meas input; theta input; psi_s1 output; ixy input; alfa3 output
function [psi_s_mag,alfa,Te,psi_s1,alfa3] = control(i_meas,theta,ixy)

% Machine parameters
ls = 0.022; % Stator inductance [H]
Lls=0.0022;
psi_r=0.5;
p=2;   % pole pairs

is_r=i_meas*(cos(theta)-1j*sin(theta));
% ids = real(is_r);
% iqs = imag(is_r);
psi_s = ls*is_r + psi_r;
psi_s1=psi_s*(cos(theta)+1j*sin(theta));
psi_s_mag=abs(psi_s1);
alfa=angle(psi_s1);
isq=imag(is_r);
Te=(5*p/2)*(psi_r*isq);
psi_xy = Lls*ixy;
% psi_xy_mag=abs(psi_xy);
alfa3=angle(psi_xy);
end

== matlab function Proposed DTC/Controller/Subsystem1/G S to v   ==
  data: v output; G input; S input
function v  = fcn(G,S)
v=1;
if (G==1)
  if (S==9) || (S==10) ||(S==1)  || (S==2) ||(S==3)
     v=1;
  elseif(S==4) || (S==5) ||(S==6)  || (S==7) ||(S==8)
     v=11;
  end
elseif (G==2)
  if (S==2) || (S==3) ||(S==4)  || (S==5) ||(S==6)
     v=2;
  elseif(S==7) || (S==8) ||(S==9)  || (S==10) ||(S==1)
     v=12;
  end
elseif (G==3)
  if (S==5) || (S==6) ||(S==7)  || (S==8) ||(S==9)
     v=3;
  elseif(S==10) || (S==1) ||(S==2)  || (S==3) ||(S==4)
     v=13;
  end
elseif (G==4)
  if (S==8) || (S==9) ||(S==10)  || (S==1) ||(S==2)
     v=4;
  elseif(S==3) || (S==4) ||(S==5)  || (S==6) ||(S==7)
     v=14;
  end
elseif (G==5)
  if (S==1) || (S==2) ||(S==3)  || (S==4) ||(S==5)
     v=5;
  elseif(S==6) || (S==7) ||(S==8)  || (S==9) ||(S==10)
     v=15;
  end  
elseif (G==6)
  if (S==4) || (S==5) ||(S==6)  || (S==7) ||(S==8)
     v=6;
  elseif(S==9) || (S==10) ||(S==1)  || (S==2) ||(S==3)
     v=16;
  end
elseif (G==7)
  if (S==7) || (S==8) ||(S==9)  || (S==10) ||(S==1)
     v=7;
  elseif(S==2) || (S==3) ||(S==4)  || (S==5) ||(S==6)
     v=17;
  end
elseif (G==8)
  if (S==10) || (S==1) ||(S==2)  || (S==3) ||(S==4)
     v=8;
  elseif (S==5) ||(S==6)  || (S==7) ||(S==8)|| (S==9)
     v=18;
  end
elseif (G==9)
  if (S==3) || (S==4) ||(S==5)  || (S==6) ||(S==7)
     v=9;
  elseif(S==8) || (S==9) ||(S==10)  || (S==1) ||(S==2)
     v=19;
  end  
elseif(G==10)
  if (S==6) || (S==7) ||(S==8)  || (S==9) ||(S==10)
     v=10;
  elseif(S==1) || (S==2) || (S==3) ||(S==4)  || (S==5)
     v=20;
  end
else
    v=0;
end

== matlab function Proposed DTC/Controller/Subsystem1/v to G ==
  data: v input; G output
function G  = fcn(v)
% low speed of operation
if (v==1) || (v==11) ||(v==21) 
     G=1;
elseif(v==2) || (v==12) ||(v==22) 
     G=2;
elseif(v==3) || (v==13) ||(v==23) 
     G=3;
 elseif(v==4) ||(v==14) ||(v==24) 
     G=4;   
 elseif(v==5) || (v==15) ||(v==25) 
     G=5;   
elseif(v==6) || (v==16) ||(v==26) 
     G=6;
elseif(v==7) || (v==17) ||(v==27) 
     G=7;
elseif(v==8) || (v==18) ||(v==28) 
     G=8;
elseif(v==9) || (v==19) ||(v==29) 
     G=9;
elseif(v==10) || (v==20) ||(v==30) 
     G=10;
else
    G=11;
end

== matlab function Proposed DTC/Controller/Sector Identification ==
  data: theta input; n output
function n  = control(theta)
alfa = (180/pi)*theta;
n=1;
if alfa<18 && alfa>0
    n=1;
elseif alfa>18 && alfa<36
    n=2;
elseif alfa>36 && alfa<54
    n=3;
elseif alfa>54 && alfa<72
    n=4;
elseif alfa>72 && alfa<90
    n=5;
elseif alfa>90 && alfa<108
    n=6;
elseif alfa>108 && alfa<126
    n=7;    
elseif alfa>126 && alfa<144
    n=8;    
elseif alfa>144 && alfa<162
    n=9;    
elseif alfa>162 && alfa<180
    n=10;       
elseif alfa>-180 && alfa<-162
    n=11;
elseif alfa>-162 && alfa<-144
    n=12;
elseif  alfa>-144 && alfa<-126
    n=13;
elseif alfa>-126 && alfa<-108
    n=14;
elseif alfa>-108 && alfa<-90
    n=15;
elseif  alfa>-90 && alfa<-72
    n=16;
elseif  alfa>-72 && alfa<-54
    n=17;
elseif  alfa>-54 && alfa<-36
    n=18;
elseif  alfa>-36 && alfa<-18
    n=19;
elseif  alfa>-18 && alfa<0
    n=20;
end
end
